simulink model "P3_Modelo_4_6_EncodersCuadratura"  (R2021b)
settings: Solver=VariableStepAuto  StartTime=0.0  StopTime=10.0  RelTol=1e-3
model workspace (MAT data in the model file):
  K = 1
settings Model: Creator=Pc24  LastModifiedBy=Pc24

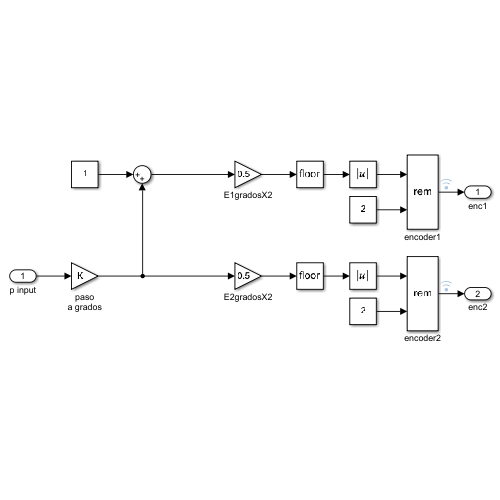
[thumbnail: Simulink's stored preview of the top-level diagram]
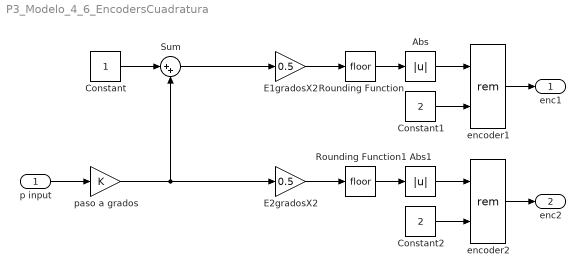
== system P3_Modelo_4_6_EncodersCuadratura ==
  p input : Inport
  Abs : Abs
  Abs1 : Abs
  Constant : Constant
  Constant1 : Constant  Value=2
  Constant2 : Constant  Value=2
  E1gradosX2 : Gain  Gain=0.5
  E2gradosX2 : Gain  Gain=0.5
  Rounding Function : Rounding
  Rounding Function1 : Rounding
  Sum : Sum  Inputs=|++
  encoder1 : Math  Operator=rem  SaturateOnIntegerOverflow=on
  encoder2 : Math  Operator=rem  SaturateOnIntegerOverflow=on
  paso a grados : Gain  Gain=K
  enc1 : Outport
  enc2 : Outport  Port=2
  wires:
  p input/1 -> paso a grados/1
  Constant/1 -> Sum/1
  paso a grados/1 -> E2gradosX2/1, Sum/2
  Sum/1 -> E1gradosX2/1
  E2gradosX2/1 -> Rounding Function1/1
  E1gradosX2/1 -> Rounding Function/1
  Rounding Function/1 -> Abs/1
  Rounding Function1/1 -> Abs1/1
  Abs/1 -> encoder1/1
  Constant1/1 -> encoder1/2
  encoder1/1 -> enc1/1
  Abs1/1 -> encoder2/1
  encoder2/1 -> enc2/1
  Constant2/1 -> encoder2/2
